simulink library "twoNodeTether_cl"  (R2018b)
settings: Solver=VariableStepAuto  StartTime=0.0  StopTime=10.0  RelTol=1e-3
undefined symbols (not defined in the file): thr
libraries: tetherDragForceNEqual2_ul x1, tetherInternalForcesNEqual2_ul x1
settings Model: Creator=asiddiq2  LastModifiedBy=mcobb

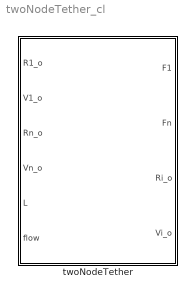
== system twoNodeTether_cl ==
  twoNodeTether : Subsystem

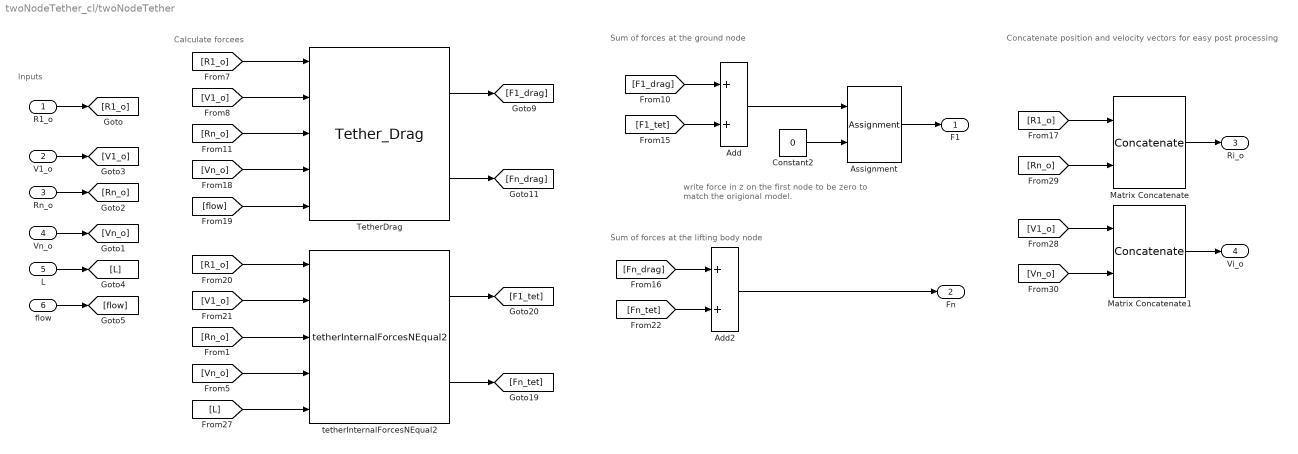
== system twoNodeTether_cl/twoNodeTether ==
  note: Concatenate position and velocity vectors for easy
      | post processing
  note: Calculate forcees
  note: Sum of forces at the lifting body node
  note: Sum of forces at the ground node
  note: write force in z on the first node to be zero
      | to match the origional model.
  note: Inputs
  R1_o : Inport
  V1_o : Inport  Port=2
  Rn_o : Inport  Port=3
  Vn_o : Inport  Port=4
  L : Inport  Port=5
  flow : Inport  Port=6
  Add : Sum
  Add2 : Sum
  Assignment : Assignment  NumberOfDimensions=2  DiagnosticForDimensions=Warning  IndexOptions=Index vector (dialog),Index vector (dialog)  Indices=3,1  OutputSizes=1,1
  Constant2 : Constant  Value=0
  Matrix Concatenate : Concatenate  Mode=Multidimensional array  ConcatenateDimension=2
  Matrix Concatenate1 : Concatenate  Mode=Multidimensional array  ConcatenateDimension=2
  TetherDrag : tetherDragForceNEqual2_ul/Tether_Drag  Cd=thr.dragCoeff  rho_fluid=fluidDensity  dia_t=thr.diameter  N=thr.numNodes
  tetherInternalForcesNEqual2 : tetherInternalForcesNEqual2_ul/tetherInternalForcesNEqual2  N=thr.numNodes  E=thr.youngsMod  dia_t=thr.diameter  mass=thr.vehicleMass  zeta=thr.dampingRatio
  F1 : Outport
  Fn : Outport  Port=2
  Ri_o : Outport  Port=3
  Vi_o : Outport  Port=4
  wires:
  R1_o/1 -> [R1_o]
  V1_o/1 -> [V1_o]
  Rn_o/1 -> [Rn_o]
  Vn_o/1 -> [Vn_o]
  L/1 -> [L]
  flow/1 -> [flow]
  [F1_drag] -> Add/1
  [F1_tet] -> Add/2
  Assignment/1 -> F1/1
  Add/1 -> Assignment/1
  Constant2/1 -> Assignment/2
  TetherDrag/1 -> [F1_drag]
  TetherDrag/2 -> [Fn_drag]
  tetherInternalForcesNEqual2/2 -> [Fn_tet]
  tetherInternalForcesNEqual2/1 -> [F1_tet]
  [Fn_drag] -> Add2/1
  [Fn_tet] -> Add2/2
  Add2/1 -> Fn/1
  [R1_o] -> TetherDrag/1
  [V1_o] -> TetherDrag/2
  [Rn_o] -> TetherDrag/3
  [Vn_o] -> TetherDrag/4
  [flow] -> TetherDrag/5
  [Rn_o] -> Matrix Concatenate/2
  [R1_o] -> Matrix Concatenate/1
  Matrix Concatenate/1 -> Ri_o/1
  [V1_o] -> Matrix Concatenate1/1
  Matrix Concatenate1/1 -> Vi_o/1
  [Vn_o] -> Matrix Concatenate1/2
  [Vn_o] -> tetherInternalForcesNEqual2/4
  [Rn_o] -> tetherInternalForcesNEqual2/3
  [V1_o] -> tetherInternalForcesNEqual2/2
  [R1_o] -> tetherInternalForcesNEqual2/1
  [L] -> tetherInternalForcesNEqual2/5
